simulink subsystem "AirspeedController"  (R2020b)
settings: Solver=VariableStepAuto  StartTime=0.0  StopTime=10.0  RelTol=1e-3
undefined symbols (not defined in the file): constr, DE2019, DiscIntNeverNeededParam, ENVMT, loiterStates, params, simInit
libraries: simulink x2
settings Model: Creator=dylaneijkelhof  LastModifiedBy=jesse

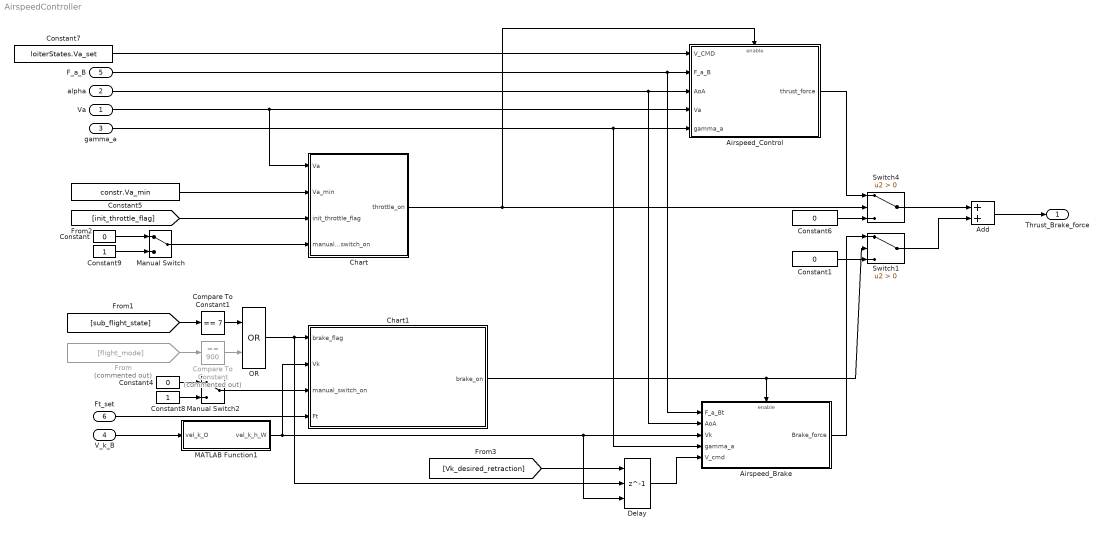
== system AirspeedController ==
  Va : Inport
  alpha : Inport  Port=2
  gamma_a : Inport  Port=3
  V_k_B : Inport  Port=4
  F_a_B : Inport  Port=5
  Ft_set : Inport  Port=6
  Add : Sum
  Airspeed_Brake : Subsystem
  Airspeed_Control : Subsystem
  Chart : Stateflow chart  TreatAsAtomicUnit=on
  Chart1 : Stateflow chart  TreatAsAtomicUnit=on  mask{Ft_retract=params.F_t_retraction_set*params.F_t_traction_set, Vk_min=30}
      mask prompts: Ft_retract "Retraction force"; Vk_min "Minimum Vk"
  Compare To Constant : simulink/Logic and Bit Operations/Compare To Constant  Commented=on  relop===  const=900  OutDataTypeStr=boolean
  Compare To Constant1 : simulink/Logic and Bit Operations/Compare To Constant  relop===  const=7  OutDataTypeStr=boolean
  Constant{,1,4,6} (4 alike) : Constant  Value=0
  Constant5 : Constant  Value=constr.Va_min
  Constant7 : Constant  Value=loiterStates.Va_set
  Constant8 : Constant
  Constant9 : Constant
  Delay : Delay  DelayLength=1  InitialConditionSource=Input port  ExternalReset=Rising
      settings: InputPortMap=u0,r5,p4
  From : From  Commented=on  GotoTag=flight_mode  TagVisibility=global
  MATLAB Function1 : MATLAB Function  TreatAsAtomicUnit=on
  Manual Switch : ManualSwitch
  Manual Switch2 : ManualSwitch
  OR : Logic  Operator=OR  IconShape=distinctive  AllPortsSameDT=off  OutDataTypeStr=boolean
  Switch1 : Switch  Criteria=u2 > Threshold
  Switch4 : Switch  Criteria=u2 > Threshold
  Thrust_Brake_force : Outport  VectorParamsAs1DForOutWhenUnconnected=off
  wires:
  Switch4/1 -> Add/1
  gamma_a/1 -> Airspeed_Brake/4(gamma_a), Airspeed_Control/5(gamma_a)
  F_a_B/1 -> Airspeed_Brake/1(F_a_Bt), Airspeed_Control/2(F_a_B)
  Constant6/1 -> Switch4/3
  Constant/1 -> Manual Switch/1
  Manual Switch/1 -> Chart/4(manual_switch_on)
  Constant7/1 -> Airspeed_Control/1(V_CMD)
  alpha/1 -> Airspeed_Brake/2(AoA), Airspeed_Control/3(AoA)
  [init_throttle_flag] -> Chart/3(init_throttle_flag)
  Constant9/1 -> Manual Switch/2
  Chart/1(throttle_on) -> Airspeed_Control/Enable, Switch4/2
  Va/1 -> Airspeed_Control/4(Va), Chart/1(Va)
  Constant5/1 -> Chart/2(Va_min)
  Airspeed_Control/1(thrust_force) -> Switch4/1
  Chart1/1(brake_on) -> Airspeed_Brake/Enable, Switch1/2
  Airspeed_Brake/1(Brake_force) -> Switch1/1
  Ft_set/1 -> Chart1/4(Ft)
  Manual Switch2/1 -> Chart1/3(manual_switch_on)
  OR/1 -> Delay/2, Chart1/1(brake_flag)
  [sub_flight_state] -> Compare To Constant1/1
  From/1 -> Compare To Constant/1
  Add/1 -> Thrust_Brake_force/1
  Constant4/1 -> Manual Switch2/1
  Constant8/1 -> Manual Switch2/2
  Delay/1 -> Airspeed_Brake/5(V_cmd)
  V_k_B/1 -> MATLAB Function1/1(vel_k_O)
  MATLAB Function1/1(vel_k_h_W) -> Airspeed_Brake/3(Vk), Delay/3, Chart1/2(Vk)
  Compare To Constant1/1 -> OR/1
  Compare To Constant/1 -> OR/2
  [Vk_desired_retraction] -> Delay/1
  Constant1/1 -> Switch1/3
  Switch1/1 -> Add/2

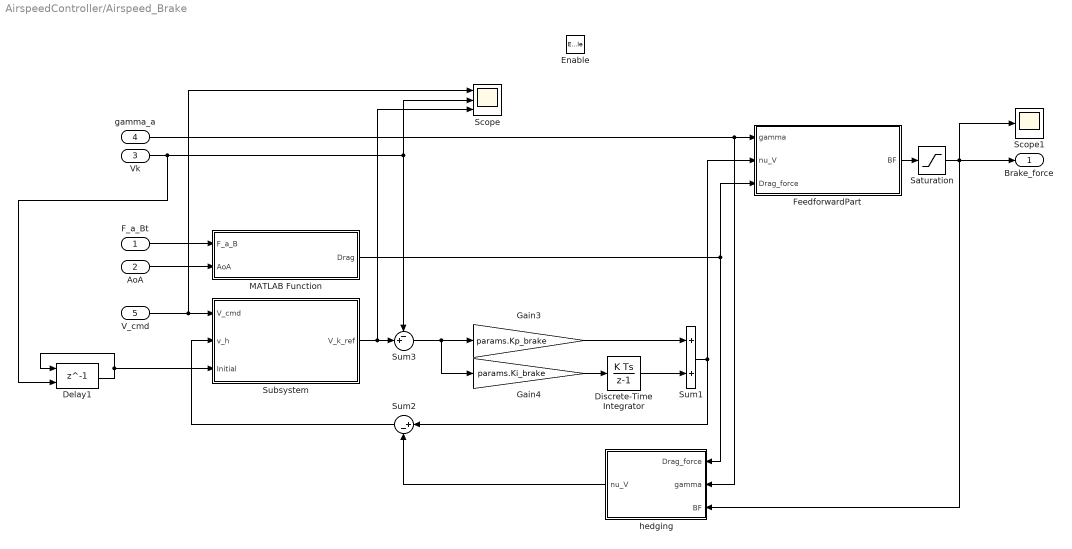
== system AirspeedController/Airspeed_Brake ==
  F_a_Bt : Inport  PortDimensions=[3,1]
  AoA : Inport  Port=2
  Vk : Inport  Port=3
  gamma_a : Inport  Port=4
  V_cmd : Inport  Port=5
  Enable : EnablePort
  Delay1 : Delay  DelayLength=1  InitialConditionSource=Input port  InitialCondition=zeros(3,1)
      settings: InputPortMap=u0,p4
  Discrete-Time Integrator : DiscreteIntegrator  SampleTime=-1  ICPrevOutput=DiscIntNeverNeededParam  ICPrevScaledInput=DiscIntNeverNeededParam
  FeedforwardPart : MATLAB Function  TreatAsAtomicUnit=on
  Gain3 : Gain  Gain=params.Kp_brake
  Gain4 : Gain  Gain=params.Ki_brake
  MATLAB Function : MATLAB Function  TreatAsAtomicUnit=on
  Saturation : Saturate  UpperLimit=0  LowerLimit=-inf  LinearizeAsGain=off
  Scope : Scope  NumInputPorts=3
  Scope1 : Scope
  Subsystem : Subsystem
  Sum1 : Sum
  Sum2 : Sum  Inputs=|+-
  Sum3 : Sum  Inputs=-+|
  hedging : MATLAB Function  TreatAsAtomicUnit=on
  Brake_force : Outport  VectorParamsAs1DForOutWhenUnconnected=off
  wires:
  Vk/1 -> Scope/2, Sum3/1, Delay1/2
  Delay1/1 -> Delay1/1, Subsystem/3(Initial)
  V_cmd/1 -> Subsystem/1(V_cmd), Scope/1
  Gain4/1 -> Discrete-Time Integrator/1
  Discrete-Time Integrator/1 -> Sum1/2
  Gain3/1 -> Sum1/1
  Sum3/1 -> Gain3/1, Gain4/1
  gamma_a/1 -> FeedforwardPart/1(gamma), hedging/2(gamma)
  Subsystem/1(V_k_ref) -> Sum3/2, Scope/3
  Sum1/1 -> FeedforwardPart/2(nu_V), Sum2/1
  Saturation/1 -> hedging/3(BF), Scope1/1, Brake_force/1
  FeedforwardPart/1(BF) -> Saturation/1
  hedging/1(nu_V) -> Sum2/2
  Sum2/1 -> Subsystem/2(v_h)
  F_a_Bt/1 -> MATLAB Function/1(F_a_B)
  MATLAB Function/1(Drag) -> hedging/1(Drag_force), FeedforwardPart/3(Drag_force)
  AoA/1 -> MATLAB Function/2(AoA)

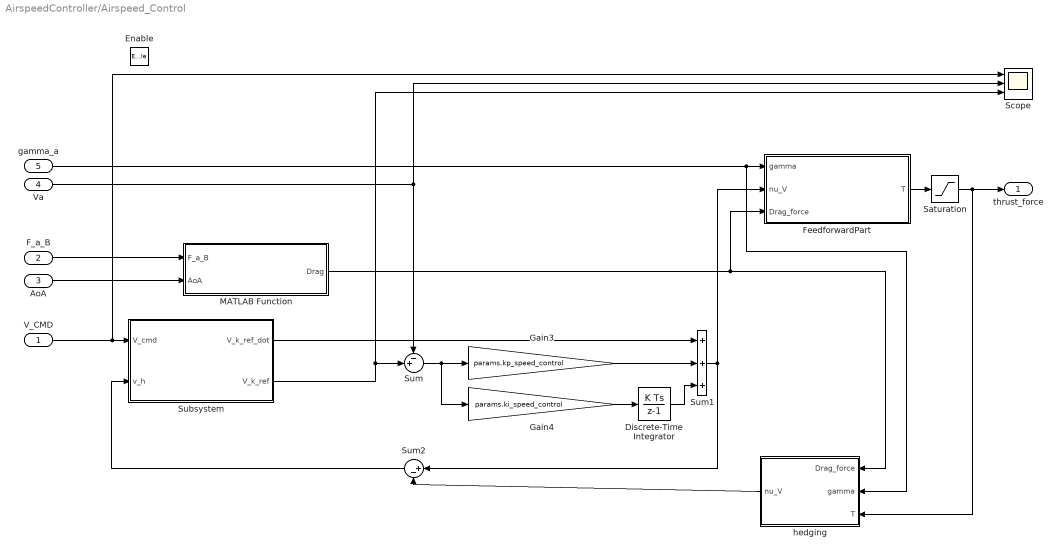
== system AirspeedController/Airspeed_Control ==
  V_CMD : Inport
  F_a_B : Inport  Port=2  PortDimensions=[3,1]
  AoA : Inport  Port=3
  Va : Inport  Port=4
  gamma_a : Inport  Port=5
  Enable : EnablePort
  Discrete-Time Integrator : DiscreteIntegrator  SampleTime=-1  ICPrevOutput=DiscIntNeverNeededParam  ICPrevScaledInput=DiscIntNeverNeededParam
  FeedforwardPart : MATLAB Function  TreatAsAtomicUnit=on
  Gain3 : Gain  Gain=params.kp_speed_control
  Gain4 : Gain  Gain=params.ki_speed_control
  MATLAB Function : MATLAB Function  TreatAsAtomicUnit=on
  Saturation : Saturate  UpperLimit=inf  LowerLimit=0  LinearizeAsGain=off
  Scope : Scope  NumInputPorts=3
  Subsystem : Subsystem
  Sum : Sum  Inputs=-+|
  Sum1 : Sum  Inputs=+++
  Sum2 : Sum  Inputs=|+-
  hedging : MATLAB Function  TreatAsAtomicUnit=on
  thrust_force : Outport  VectorParamsAs1DForOutWhenUnconnected=off
  wires:
  Gain4/1 -> Discrete-Time Integrator/1
  Discrete-Time Integrator/1 -> Sum1/3
  Gain3/1 -> Sum1/2
  Va/1 -> Sum/1, Scope/2
  Sum/1 -> Gain3/1, Gain4/1
  V_CMD/1 -> Scope/1, Subsystem/1(V_cmd)
  gamma_a/1 -> FeedforwardPart/1(gamma), hedging/2(gamma)
  Subsystem/2(V_k_ref) -> Scope/3, Sum/2
  Sum1/1 -> FeedforwardPart/2(nu_V), Sum2/1
  Subsystem/1(V_k_ref_dot) -> Sum1/1
  Saturation/1 -> hedging/3(T), thrust_force/1
  FeedforwardPart/1(T) -> Saturation/1
  hedging/1(nu_V) -> Sum2/2
  Sum2/1 -> Subsystem/2(v_h)
  F_a_B/1 -> MATLAB Function/1(F_a_B)
  MATLAB Function/1(Drag) -> FeedforwardPart/3(Drag_force), hedging/1(Drag_force)
  AoA/1 -> MATLAB Function/2(AoA)

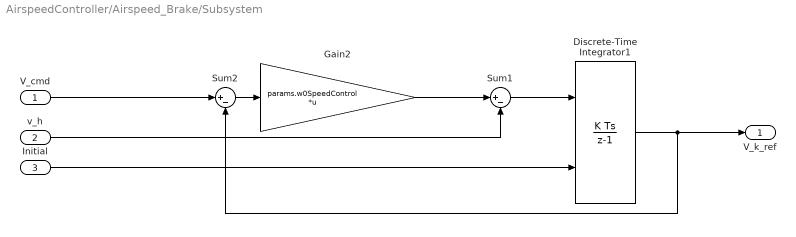
== system AirspeedController/Airspeed_Brake/Subsystem ==
  V_cmd : Inport
  v_h : Inport  Port=2
  Initial : Inport  Port=3
  Discrete-Time Integrator1 : DiscreteIntegrator  InitialConditionSource=external  InitialCondition=norm(simInit.vel_B_init)  SampleTime=-1  LimitOutput=on  UpperSaturationLimit=120  LowerSaturationLimit=0  ICPrevOutput=DiscIntNeverNeededParam  ICPrevScaledInput=DiscIntNeverNeededParam
  Gain2 : Gain  Gain=params.w0SpeedControl  Multiplication=Matrix(K*u)
  Sum1 : Sum  Inputs=|+-
  Sum2 : Sum  Inputs=|+-
  V_k_ref : Outport  VectorParamsAs1DForOutWhenUnconnected=off
  wires:
  Initial/1 -> Discrete-Time Integrator1/2
  Discrete-Time Integrator1/1 -> V_k_ref/1, Sum2/2
  Sum2/1 -> Gain2/1
  V_cmd/1 -> Sum2/1
  Sum1/1 -> Discrete-Time Integrator1/1
  v_h/1 -> Sum1/2
  Gain2/1 -> Sum1/1

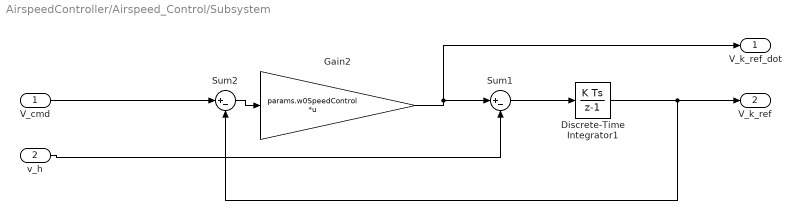
== system AirspeedController/Airspeed_Control/Subsystem ==
  V_cmd : Inport
  v_h : Inport  Port=2
  Discrete-Time Integrator1 : DiscreteIntegrator  InitialCondition=norm(simInit.vel_B_init)  SampleTime=-1  LimitOutput=on  UpperSaturationLimit=120  LowerSaturationLimit=0  ICPrevOutput=DiscIntNeverNeededParam  ICPrevScaledInput=DiscIntNeverNeededParam
  Gain2 : Gain  Gain=params.w0SpeedControl  Multiplication=Matrix(K*u)
  Sum1 : Sum  Inputs=|+-
  Sum2 : Sum  Inputs=|+-
  V_k_ref_dot : Outport  VectorParamsAs1DForOutWhenUnconnected=off
  V_k_ref : Outport  Port=2  VectorParamsAs1DForOutWhenUnconnected=off
  wires:
  Discrete-Time Integrator1/1 -> Sum2/2, V_k_ref/1
  Sum2/1 -> Gain2/1
  V_cmd/1 -> Sum2/1
  Sum1/1 -> Discrete-Time Integrator1/1
  v_h/1 -> Sum1/2
  Gain2/1 -> V_k_ref_dot/1, Sum1/1

== stateflow chart AirspeedController/Chart ==
  state Throttle_Off
    entry: throttle_on = 0;
  state Throttle_On
    entry: throttle_on = 1;
  (default) -> Throttle_Off
  Throttle_Off -> Throttle_On : [Va<Va_min || manual_switch_on || init_throttle_flag]
  Throttle_On -> Throttle_Off : [Va>Va_min+10&&manual_switch_on==0&& init_throttle_flag ==0]
  data: Va input; Va_min input; init_throttle_flag input; throttle_on output; manual_switch_on input

== stateflow chart AirspeedController/Chart1 ==
  state Throttle_Off
    entry: brake_on = 0;
  state Throttle_On
    entry: brake_on = 1;
  (default) -> Throttle_Off
  Throttle_Off -> Throttle_On : [(manual_switch_on || brake_flag) && Ft <= Ft_retract+3000 && Vk>Vk_min]
  Throttle_On -> Throttle_Off : [(manual_switch_on==0&& brake_flag ==0) || Vk<Vk_min]
  data: brake_flag input; Vk input; brake_on output; manual_switch_on input; Ft input; Ft_retract parameter; Vk_min parameter

== matlab function AirspeedController/Airspeed_Brake/FeedforwardPart ==
  data: gamma input; BF output; nu_V input; ENVMT parameter; Drag_force input; DE2019 parameter
% Copyright 2021 Delft University of Technology
%
% Licensed under the Apache License, Version 2.0 (the "License");
% you may not use this file except in compliance with the License.
% You may obtain a copy of the License at
%
%      http://www.apache.org/licenses/LICENSE-2.0
%
% Unless required by applicable law or agreed to in writing, software
% distributed under the License is distributed on an "AS IS" BASIS,
% WITHOUT WARRANTIES OR CONDITIONS OF ANY KIND, either express or implied.
% See the License for the specific language governing permissions and
% limitations under the License.

function BF = feedforward_brake(gamma, nu_V,  ENVMT, Drag_force, DE2019)
%feedforward_brake - Brake force calculation for velocity decrease
%
% Inputs:
%    gamma      - Path angle (glideslope)
%    nu_V       - Controlled velocity parameter
%    ENVMT      - Environmental characteristics
%    Drag_force	- Drag
%    DE2019     - Aircraft characteristics
%
% Outputs:
%    BF          - Brake force
%
% Example: 
%    BF = feedforward_thrust(gamma, nu_V,  ENVMT, Drag_force, DE2019)
%
% Author: Sebastian Rapp, Ph.D., Revised by: Dylan Eijkelhof, M.Sc.
% Delft University of Technology
% email address: s.rapp@tudelft.nl
% email address: d.eijkelhof@tudelft.nl
% December 2019; Last revision: 06-October-2020

%-------------	BEGIN CODE	--------------

BF = DE2019.mass * ( ENVMT.g * sin(gamma) + nu_V ) + Drag_force; % required thrust

%-------------	 END CODE	--------------
end

== matlab function AirspeedController/Airspeed_Brake/MATLAB Function ==
  data: F_a_B input; Drag output; AoA input
% Copyright 2021 Delft University of Technology
%
% Licensed under the Apache License, Version 2.0 (the "License");
% you may not use this file except in compliance with the License.
% You may obtain a copy of the License at
%
%      http://www.apache.org/licenses/LICENSE-2.0
%
% Unless required by applicable law or agreed to in writing, software
% distributed under the License is distributed on an "AS IS" BASIS,
% WITHOUT WARRANTIES OR CONDITIONS OF ANY KIND, either express or implied.
% See the License for the specific language governing permissions and
% limitations under the License.

function Drag  = estimate_drag(F_a_B, AoA)
%estimate_drag - Transform drag from B to A reference frame
%
% Inputs:
%    F_a_B     - Aerodynamic forces in body reference frame
%    AoA       - Angle of Attack
%
% Outputs:
%    Drag    - Drag force
%
% Example: 
%    [Drag] = estimate_drag(F_a_B, AoA)
%
% Author: Sebastian Rapp, Ph.D., Revised by: Dylan Eijkelhof, M.Sc.
% Delft University of Technology
% email address: s.rapp@tudelft.nl
% email address: d.eijkelhof@tudelft.nl
% December 2019; Last revision: 06-October-2020

%-------------	BEGIN CODE	--------------

F_a_A = [cos(AoA), 0, sin(AoA);
    0, 1, 0; 
    -sin(AoA), 0, cos(AoA)] * F_a_B;

Drag = -F_a_A(1);

%-------------	 END CODE	--------------

end

== matlab function AirspeedController/Airspeed_Brake/hedging ==
  data: Drag_force input; gamma input; nu_V output; BF input; ENVMT parameter; DE2019 parameter
% Copyright 2021 Delft University of Technology
%
% Licensed under the Apache License, Version 2.0 (the "License");
% you may not use this file except in compliance with the License.
% You may obtain a copy of the License at
%
%      http://www.apache.org/licenses/LICENSE-2.0
%
% Unless required by applicable law or agreed to in writing, software
% distributed under the License is distributed on an "AS IS" BASIS,
% WITHOUT WARRANTIES OR CONDITIONS OF ANY KIND, either express or implied.
% See the License for the specific language governing permissions and
% limitations under the License.

function nu_V = hedgingV(Drag_force, gamma, BF, ENVMT, DE2019)

%hedgingV
%
% Inputs:
%    Drag_force	- Drag
%    gamma      - Path angle (glideslope)
%    BF         - Brake force
%    ENVMT      - Environmental characteristics
%    DE2019     - Aircraft characteristics
%
% Outputs:
%    nu_V       - Controlled velocity parameter
%
% Example: 
%    nu_V = hedgingV(Drag_force, gamma, BF, ENVMT, DE2019)
%
% Author: Sebastian Rapp, Ph.D., Revised by: Dylan Eijkelhof, M.Sc.
% Delft University of Technology
% email address: s.rapp@tudelft.nl
% email address: d.eijkelhof@tudelft.nl
% December 2019; Last revision: 06-October-2020

%-------------	BEGIN CODE	--------------

nu_V = (BF-Drag_force)/DE2019.mass - ENVMT.g * sin(gamma); 

%-------------	 END CODE	--------------
end

== matlab function AirspeedController/MATLAB Function1 ==
  data: vel_k_O input; vel_k_h_W output; ENVMT parameter
% Copyright 2021 Delft University of Technology
%
% Licensed under the Apache License, Version 2.0 (the "License");
% you may not use this file except in compliance with the License.
% You may obtain a copy of the License at
%
%      http://www.apache.org/licenses/LICENSE-2.0
%
% Unless required by applicable law or agreed to in writing, software
% distributed under the License is distributed on an "AS IS" BASIS,
% WITHOUT WARRANTIES OR CONDITIONS OF ANY KIND, either express or implied.
% See the License for the specific language governing permissions and
% limitations under the License.

function vel_k_h_W    = fcn(vel_k_O,ENVMT)
%fcn - Calculate horizontal kinetic velocity in wind reference frame
%
% Inputs:
%    vel_k_O    - Kinetic velocity in inertial reference frame
%    ENVMT      - Environment characteristics
%
% Outputs:
%    vel_k_h_W  - Horizontal kinetic velocity magnitude in wind reference frame
%
%
% Author: Sebastian Rapp, Ph.D., Revised by: Dylan Eijkelhof, M.Sc.
% Delft University of Technology
% email address: s.rapp@tudelft.nl
% email address: d.eijkelhof@tudelft.nl
% December 2019; Last revision: 06-October-2020

%-------------	BEGIN CODE	--------------

vel_k_W = transformFromOtoW(ENVMT.windDirection_rad, vel_k_O);

vel_k_h_W = sign(-vel_k_W(1))*sqrt( vel_k_W(1)^2 + vel_k_W(2)^2 );

%-------------	 END CODE	--------------
end

== matlab function AirspeedController/Airspeed_Control/FeedforwardPart ==
  data: gamma input; T output; nu_V input; ENVMT parameter; Drag_force input; DE2019 parameter
% Copyright 2021 Delft University of Technology
%
% Licensed under the Apache License, Version 2.0 (the "License");
% you may not use this file except in compliance with the License.
% You may obtain a copy of the License at
%
%      http://www.apache.org/licenses/LICENSE-2.0
%
% Unless required by applicable law or agreed to in writing, software
% distributed under the License is distributed on an "AS IS" BASIS,
% WITHOUT WARRANTIES OR CONDITIONS OF ANY KIND, either express or implied.
% See the License for the specific language governing permissions and
% limitations under the License.

function T = feedforward_thrust(gamma, nu_V,  ENVMT, Drag_force, DE2019)
%feedforward_thrust - Thrust calculation for velocity initialisation
%
% Inputs:
%    gamma      - Path angle (glideslope)
%    nu_V       - Controlled velocity parameter
%    ENVMT      - Environmental characteristics
%    Drag_force	- Drag
%    DE2019     - Aircraft characteristics
%
% Outputs:
%    T          - Thrust force
%
% Example: 
%    T = feedforward_thrust(gamma, nu_V,  ENVMT, Drag_force, DE2019)
%
% Author: Sebastian Rapp, Ph.D., Revised by: Dylan Eijkelhof, M.Sc.
% Delft University of Technology
% email address: s.rapp@tudelft.nl
% email address: d.eijkelhof@tudelft.nl
% December 2019; Last revision: 06-October-2020

%-------------	BEGIN CODE	--------------

T = DE2019.mass * ( ENVMT.g * sin(gamma) + nu_V ) + Drag_force; % required thrust

% Based on the quotient of commmanded to max. available thrust
% F_T_max = ENVMT.rhos * DE2019.S_prop * DE2019.C_prop * DE2019.k_motor * (DE2019.k_motor - Va);
% delta_t = T/F_T_max; 

%-------------	 END CODE	--------------
end

== matlab function AirspeedController/Airspeed_Control/MATLAB Function ==
  data: F_a_B input; Drag output; AoA input
% Copyright 2021 Delft University of Technology
%
% Licensed under the Apache License, Version 2.0 (the "License");
% you may not use this file except in compliance with the License.
% You may obtain a copy of the License at
%
%      http://www.apache.org/licenses/LICENSE-2.0
%
% Unless required by applicable law or agreed to in writing, software
% distributed under the License is distributed on an "AS IS" BASIS,
% WITHOUT WARRANTIES OR CONDITIONS OF ANY KIND, either express or implied.
% See the License for the specific language governing permissions and
% limitations under the License.

function Drag = estimate_drag(F_a_B, AoA)

%estimate_drag - Transform drag from B to A reference frame
%
% Inputs:
%    F_a_B     - Aerodynamic forces in body reference frame
%    AoA       - Angle of Attack
%
% Outputs:
%    Drag    - Drag force
%
% Example: 
%    Drag = estimate_drag(F_a_B, AoA)
%
% Author: Sebastian Rapp, Ph.D., Revised by: Dylan Eijkelhof, M.Sc.
% Delft University of Technology
% email address: s.rapp@tudelft.nl
% email address: d.eijkelhof@tudelft.nl
% December 2019; Last revision: 06-October-2020

%-------------	BEGIN CODE	--------------

F_a_A = [cos(AoA), 0, sin(AoA);
    0, 1, 0; 
    -sin(AoA), 0, cos(AoA)] * F_a_B;

Drag = -F_a_A(1);

%-------------	 END CODE	--------------
end

== matlab function AirspeedController/Airspeed_Control/hedging ==
  data: Drag_force input; gamma input; nu_V output; T input; ENVMT parameter; DE2019 parameter
% Copyright 2021 Delft University of Technology
%
% Licensed under the Apache License, Version 2.0 (the "License");
% you may not use this file except in compliance with the License.
% You may obtain a copy of the License at
%
%      http://www.apache.org/licenses/LICENSE-2.0
%
% Unless required by applicable law or agreed to in writing, software
% distributed under the License is distributed on an "AS IS" BASIS,
% WITHOUT WARRANTIES OR CONDITIONS OF ANY KIND, either express or implied.
% See the License for the specific language governing permissions and
% limitations under the License.

function nu_V = hedgingV(Drag_force, gamma, T, ENVMT, DE2019)

%hedgingV
%
% Inputs:
%    Drag_force	- Drag
%    gamma      - Path angle (glideslope)
%    T          - Thrust force
%    ENVMT      - Environmental characteristics
%    DE2019     - Aircraft characteristics
%
% Outputs:
%    nu_V       - Controlled velocity parameter
%
% Example: 
%    nu_V = hedgingV(Drag_force, gamma, T, ENVMT, DE2019)
%
% Author: Sebastian Rapp, Ph.D., Revised by: Dylan Eijkelhof, M.Sc.
% Delft University of Technology
% email address: s.rapp@tudelft.nl
% email address: d.eijkelhof@tudelft.nl
% December 2019; Last revision: 06-October-2020

%-------------	BEGIN CODE	--------------

% Based on the quotient of commmanded to max. available thrust
% F_T_max = ENVMT.rhos * DE2019.S_prop * DE2019.C_prop * DE2019.k_motor * (DE2019.k_motor - Va);
% T = F_T_max * delta_t; 

nu_V = (T-Drag_force)/DE2019.mass - ENVMT.g * sin(gamma); 

%-------------	 END CODE	--------------
end
